simulink model "ex 1"  (R2021b)
settings: Solver=VariableStepAuto  StartTime=0.0  StopTime=20.0  RelTol=1e-3
settings Model: Creator=macbook  LastModifiedBy=macbook

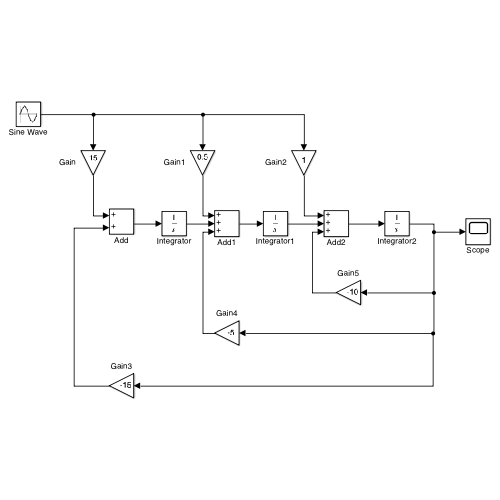
[thumbnail: Simulink's stored preview of the top-level diagram]
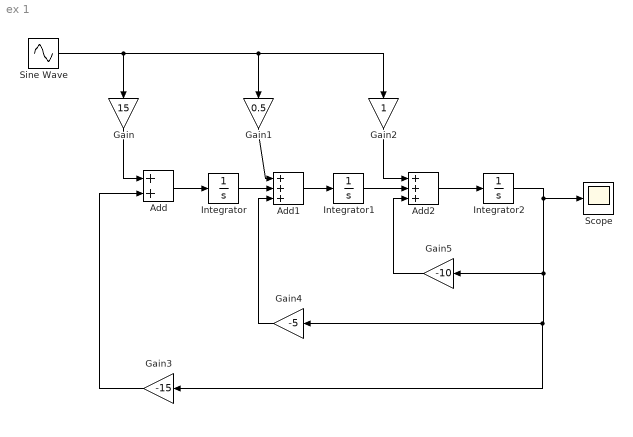
== system ex 1 ==
  Add : Sum
  Add1 : Sum  Inputs=+++
  Add2 : Sum  Inputs=+++
  Gain : Gain  Gain=15
  Gain1 : Gain  Gain=0.5
  Gain2 : Gain
  Gain3 : Gain  Gain=-15
  Gain4 : Gain  Gain=-5
  Gain5 : Gain  Gain=-10
  Integrator : Integrator  InitialCondition=10.1
  Integrator1 : Integrator  InitialCondition=10.5
  Integrator2 : Integrator  InitialCondition=1
  Scope : Scope
  Sine Wave : Sin  SampleTime=0
  wires:
  Sine Wave/1 -> Gain2/1, Gain1/1, Gain/1
  Gain/1 -> Add/1
  Add/1 -> Integrator/1
  Integrator/1 -> Add1/2
  Gain1/1 -> Add1/1
  Add1/1 -> Integrator1/1
  Add2/1 -> Integrator2/1
  Integrator1/1 -> Add2/2
  Gain2/1 -> Add2/1
  Gain3/1 -> Add/2
  Gain4/1 -> Add1/3
  Gain5/1 -> Add2/3
  Integrator2/1 -> Scope/1, Gain3/1, Gain4/1, Gain5/1
